simulink model "omega_simulink_verify"  (R2018a)
settings: Solver=VariableStepAuto  StartTime=0.0  StopTime=200  RelTol=1e-3
model workspace: external: MAT-File /home/owen/Desktop/play_ground/src/system_identification_car/scripts/matlab_omega_control/all_current_ws.mat (data not in the file)
undefined symbols (not defined in the file or in its folder): discrete_ss1, discrete_steering, K_inf, Ts
libraries: simulink x1
settings Model: Creator=root  LastModifiedBy=root

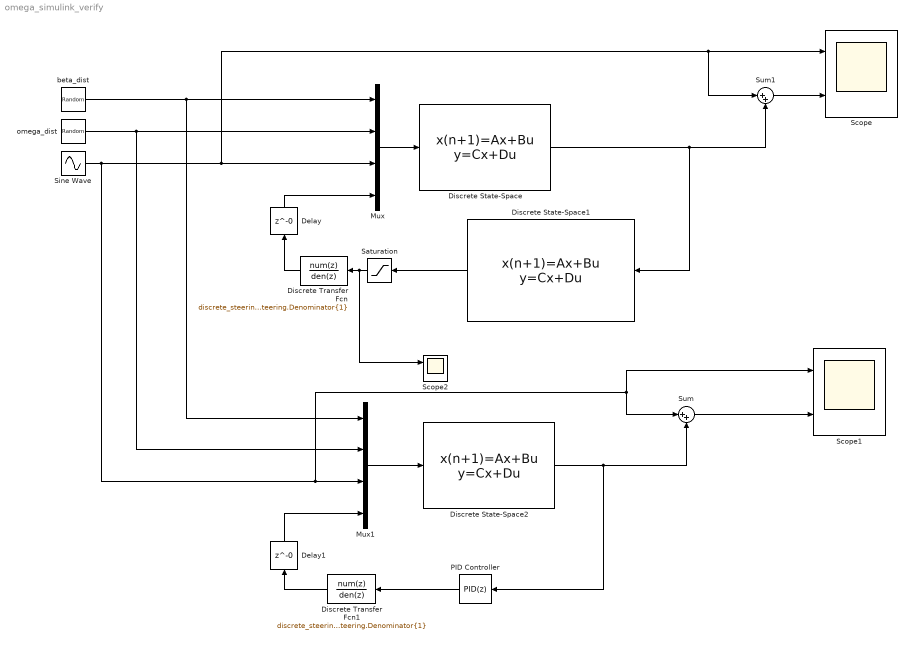
== system omega_simulink_verify ==
  Delay : Delay  DelayLength=0  SampleTime=Ts
  Delay1 : Delay  DelayLength=0  SampleTime=Ts
  Discrete Transfer Fcn : DiscreteTransferFcn  Numerator=discrete_steering.Numerator{1}  Denominator=discrete_steering.Denominator{1}  SampleTime=Ts
  Discrete Transfer Fcn1 : DiscreteTransferFcn  Numerator=discrete_steering.Numerator{1}  Denominator=discrete_steering.Denominator{1}  SampleTime=Ts
  Discrete State-Space : DiscreteStateSpace  A=discrete_ss1.A  B=discrete_ss1.B  C=discrete_ss1.C  D=discrete_ss1.D  SampleTime=Ts
  Discrete State-Space1 : DiscreteStateSpace  A=K_inf.A  B=K_inf.B  C=K_inf.C  D=K_inf.D  SampleTime=Ts
  Discrete State-Space2 : DiscreteStateSpace  A=discrete_ss1.A  B=discrete_ss1.B  C=discrete_ss1.C  D=discrete_ss1.D  SampleTime=Ts
  Mux : Mux
  Mux1 : Mux
  PID Controller : simulink/Continuous/PID Controller  Controller=PID  TimeDomain=Discrete-time  SampleTime=Ts  IntegratorMethod=Forward Euler  FilterMethod=Forward Euler  Form=Parallel  UseFilter=off  ControllerParametersSource=internal  P=-3.4  I=-3.1  D=-0.91  N=44.0888341160424  InitialConditionSource=internal  InitialConditionForIntegrator=0  InitialConditionForFilter=0  ExternalReset=none  LimitOutput=on  UpperSaturationLimit=4  LowerSaturationLimit=-4  LinearizeAsGain=off  AntiWindupMode=none  Kb=1  TrackingMode=off  Kt=1  PParamMin=[]  PParamMax=[]  IParamMin=[]  IParamMax=[]  DParamMin=[]  DParamMax=[]  NParamMin=[]  NParamMax=[]  KbParamMin=[]  KbParamMax=[]  KtParamMin=[]  KtParamMax=[]  POutMin=[]  POutMax=[]  IOutMin=[]  IOutMax=[]  DOutMin=[]  DOutMax=[]  NOutMin=[]  NOutMax=[]  KbOutMin=[]  KbOutMax=[]  KtOutMin=[]  KtOutMax=[]  IntegratorOutMin=[]  IntegratorOutMax=[]  FilterOutMin=[]  FilterOutMax=[]  SumOutMin=[]  SumOutMax=[]  SumI1OutMin=[]  SumI1OutMax=[]  SumI2OutMin=[]  SumI2OutMax=[]  SumI3OutMin=[]  SumI3OutMax=[]  SumDOutMin=[]  SumDOutMax=[]  SaturationOutMin=[]  SaturationOutMax=[]  IntegratorContinuousStateAttributes=''  IntegratorStateMustResolveToSignalObject=off  IntegratorRTWStateStorageClass=Auto  FilterContinuousStateAttributes=''  FilterStateMustResolveToSignalObject=off  FilterRTWStateStorageClass=Auto  DifferentiatorICPrevScaledInput=0  DifferentiatorOutMin=[]  DifferentiatorOutMax=[]  FilterDiffOutCoefMin=[]  FilterDiffOutCoefMax=[]  SumDenOutMin=[]  SumDenOutMax=[]  SumNumOutMin=[]  SumNumOutMax=[]  ReciprocalOutMin=[]  ReciprocalOutMax=[]  DivideOutMin=[]  DivideOutMax=[]  TunerSelectOption=Transfer Function Based (PID Tuner App)
  Saturation : Saturate  UpperLimit=4  LowerLimit=-4
  Scope : Scope  NumInputPorts=2
  Scope1 : Scope  NumInputPorts=2
  Scope2 : Scope  NumInputPorts=2
  Sine Wave : Sin  Frequency=0.4  SampleTime=0
  Sum : Sum  Inputs=|++
  Sum1 : Sum  Inputs=|++
  "beta_dist " : RandomNumber  Variance=0  Seed=1421  SampleTime=2
  omega_dist : RandomNumber  Variance=0  Seed=1231421  SampleTime=2.5
  wires:
  Mux/1 -> Discrete State-Space/1
  omega_dist/1 -> Mux1/2, Mux/2
  "beta_dist "/1 -> Mux1/1, Mux/1
  Discrete State-Space2/1 -> PID Controller/1, Sum/2
  Mux1/1 -> Discrete State-Space2/1
  Saturation/1 -> Scope2/1, Discrete Transfer Fcn/1
  Discrete Transfer Fcn/1 -> Delay/1
  Discrete Transfer Fcn1/1 -> Delay1/1
  Discrete State-Space/1 -> Discrete State-Space1/1, Sum1/2
  Discrete State-Space1/1 -> Saturation/1
  Delay/1 -> Mux/4
  Sine Wave/1 -> Scope1/1, Sum/1, Mux1/3, Sum1/1, Scope/1, Mux/3
  Delay1/1 -> Mux1/4
  Sum/1 -> Scope1/2
  Sum1/1 -> Scope/2
  PID Controller/1 -> Discrete Transfer Fcn1/1
